simulink model "port_test_B_2015B"  (R2015b)
settings: Solver=VariableStepAuto  StartTime=0.0  StopTime=10  RelTol=1e-3
libraries: dspnetwork x4, sldrtlib x1
settings Model: Creator=dave  LastModifiedBy=Anony

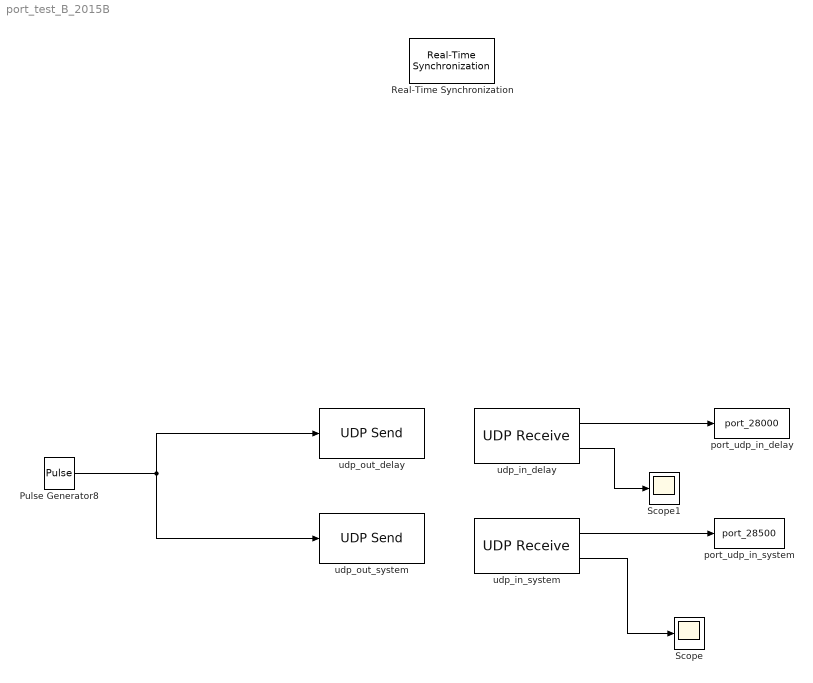
== system port_test_B_2015B ==
  Pulse Generator8 : DiscretePulseGenerator  PulseType=Time based  Period=1  PulseWidth=5
  Real-Time Synchronization : sldrtlib/Real-Time Synchronization  SampleTime=0.1  MaxMissedTicks=inf  ShowMissedTicks=off  YieldWhenWaiting=off
  Scope : Scope
  Scope1 : Scope
  port_udp_in_delay : ToWorkspace  VariableName=port_28000  SaveFormat=Timeseries  SampleTime=-1
  port_udp_in_system : ToWorkspace  VariableName=port_28500  SaveFormat=Timeseries  SampleTime=-1
  udp_in_delay : dspnetwork/UDP Receive  localURL='0.0.0.0'  localPort=28000  remoteURL='147.32.161.72'  remotePort=-1  recvBufferSize=8192  dims=255  signalDatatype=int8  isVarSize=off  showBlockingTime=off  blockingTime=0  sampletime=0.1
  udp_in_system : dspnetwork/UDP Receive  localURL='0.0.0.0'  localPort=28500  remoteURL='147.32.161.72'  remotePort=-1  recvBufferSize=8192  dims=255  signalDatatype=int8  isVarSize=off  showBlockingTime=off  blockingTime=0  sampletime=0.1
  udp_out_delay : dspnetwork/UDP Send  remoteURL='147.32.161.72'  remotePort=27000  localURL='0.0.0.0'  localPortSource=Automatically determine  localPort=-1  sampletime=-1  separateLengthPort=0
  udp_out_system : dspnetwork/UDP Send  remoteURL='147.32.161.72'  remotePort=27500  localURL='0.0.0.0'  localPortSource=Automatically determine  localPort=-1  sampletime=-1  separateLengthPort=0
  wires:
  Pulse Generator8/1 -> udp_out_delay/1, udp_out_system/1
  udp_in_system/1 -> port_udp_in_system/1
  udp_in_delay/1 -> port_udp_in_delay/1
  udp_in_system/2 -> Scope/1
  udp_in_delay/2 -> Scope1/1
